simulink model "hoverAlic"  (R2017b)
settings: Solver=VariableStepAuto  StartTime=0.0  StopTime=inf  RelTol=1e-3
values from neighbouring files (symbols this model uses):
  imu = rossubscriber('/imu')    [identification.m]
undefined symbols (not defined in the file or in its folder): Angular, Linear
libraries: robotlib x3, simulink x3
settings Model: Creator=alic  LastModifiedBy=alic

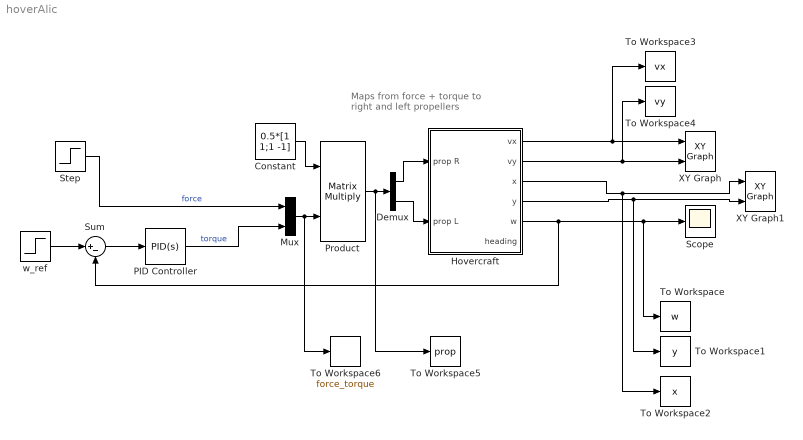
== system hoverAlic ==
  note: Maps from force + torque to
      | right and left propellers
  Constant : Constant  Value=0.5*[1 1;1 -1]
  Demux : Demux  Outputs=2
  Hovercraft : Subsystem
  Mux : Mux  Inputs=2
  PID Controller : simulink/Continuous/PID Controller  Controller=PID  TimeDomain=Continuous-time  SampleTime=-1  IntegratorMethod=Forward Euler  FilterMethod=Forward Euler  Form=Ideal  UseFilter=on  ControllerParametersSource=internal  P=-1.30263726087134  I=1.05750099590497  D=0  N=100  InitialConditionSource=internal  InitialConditionForIntegrator=0  InitialConditionForFilter=0  ExternalReset=none  LimitOutput=off  UpperSaturationLimit=inf  LowerSaturationLimit=-inf  LinearizeAsGain=on  AntiWindupMode=none  Kb=1  TrackingMode=off  Kt=1  PParamMin=[]  PParamMax=[]  IParamMin=[]  IParamMax=[]  DParamMin=[]  DParamMax=[]  NParamMin=[]  NParamMax=[]  KbParamMin=[]  KbParamMax=[]  KtParamMin=[]  KtParamMax=[]  POutMin=[]  POutMax=[]  IOutMin=[]  IOutMax=[]  DOutMin=[]  DOutMax=[]  NOutMin=[]  NOutMax=[]  KbOutMin=[]  KbOutMax=[]  KtOutMin=[]  KtOutMax=[]  IntegratorOutMin=[]  IntegratorOutMax=[]  FilterOutMin=[]  FilterOutMax=[]  SumOutMin=[]  SumOutMax=[]  SumI1OutMin=[]  SumI1OutMax=[]  SumI2OutMin=[]  SumI2OutMax=[]  SumI3OutMin=[]  SumI3OutMax=[]  SumDOutMin=[]  SumDOutMax=[]  SaturationOutMin=[]  SaturationOutMax=[]  IntegratorContinuousStateAttributes=''  IntegratorStateMustResolveToSignalObject=off  IntegratorRTWStateStorageClass=Auto  FilterContinuousStateAttributes=''  FilterStateMustResolveToSignalObject=off  FilterRTWStateStorageClass=Auto  DifferentiatorICPrevScaledInput=0  DifferentiatorOutMin=[]  DifferentiatorOutMax=[]  InitialConditionSetting=State (most efficient)  FilterDiffOutCoefMin=[]  FilterDiffOutCoefMax=[]  SumDenOutMin=[]  SumDenOutMax=[]  SumNumOutMin=[]  SumNumOutMax=[]  ReciprocalOutMin=[]  ReciprocalOutMax=[]  DivideOutMin=[]  DivideOutMax=[]  TunerSelectOption=Transfer Function Based (PID Tuner App)
  Product : Product  Multiplication=Matrix(*)
  Scope : Scope
  Step : Step  After=0.2  SampleTime=3
  Sum : Sum  Inputs=|+-
  To Workspace : ToWorkspace  VariableName=w  SaveFormat=Timeseries  SampleTime=-1
  To Workspace1 : ToWorkspace  VariableName=y  SaveFormat=Timeseries  SampleTime=-1
  To Workspace2 : ToWorkspace  VariableName=x  SaveFormat=Timeseries  SampleTime=-1
  To Workspace3 : ToWorkspace  VariableName=vx  SaveFormat=Timeseries  SampleTime=-1
  To Workspace4 : ToWorkspace  VariableName=vy  SaveFormat=Timeseries  SampleTime=-1
  To Workspace5 : ToWorkspace  VariableName=prop  SaveFormat=Timeseries  SampleTime=-1
  To Workspace6 : ToWorkspace  VariableName=force_torque  SaveFormat=Timeseries  SampleTime=-1
  XY Graph : simulink/Sinks/XY Graph  xmin=-2  xmax=2  ymin=-2  ymax=2  st=-1
  XY Graph1 : simulink/Sinks/XY Graph  xmin=-10  xmax=10  ymin=-10  ymax=10  st=-1
  w_ref : Step  After=0  SampleTime=0
  wires:
  Hovercraft/2(vy) -> To Workspace4/1, XY Graph/2
  Step/1 -> Mux/1  "force"
  Hovercraft/5(w) -> Sum/2, To Workspace/1, Scope/1
  Hovercraft/1(vx) -> To Workspace3/1, XY Graph/1
  Constant/1 -> Product/1
  w_ref/1 -> Sum/1
  Product/1 -> To Workspace5/1, Demux/1
  Mux/1 -> To Workspace6/1, Product/2
  Sum/1 -> PID Controller/1
  Hovercraft/4(y) -> To Workspace1/1, XY Graph1/2
  PID Controller/1 -> Mux/2  "torque"
  Demux/1 -> Hovercraft/1(prop R)
  Hovercraft/3(x) -> To Workspace2/1, XY Graph1/1
  Demux/2 -> Hovercraft/2(prop L)

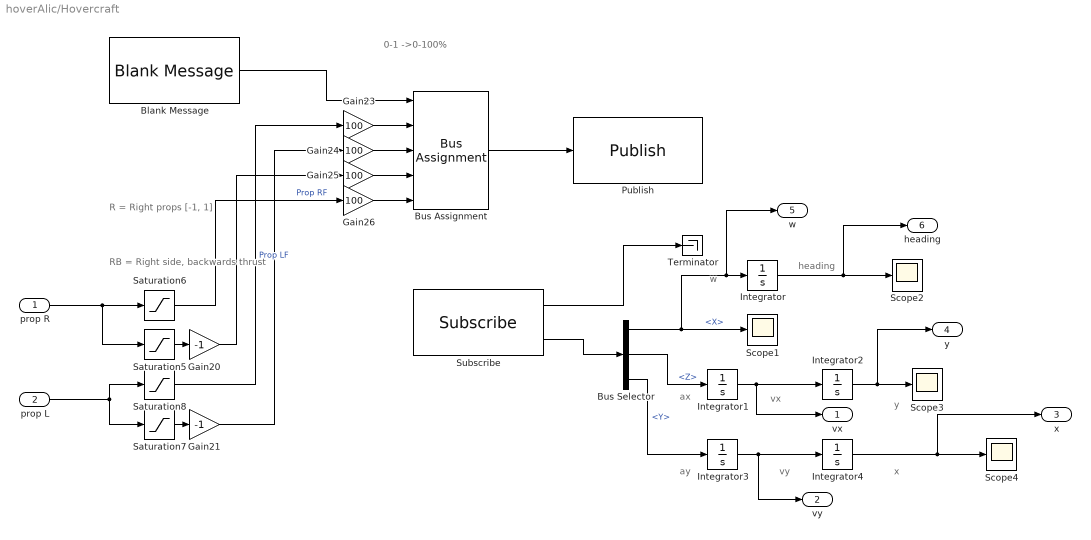
== system hoverAlic/Hovercraft ==
  note: vx
  note: ax
  note: heading
  note: w
  note: 0-1 ->0-100%
  note: R = Right props [-1, 1]
  note: RB = Right side, backwards thrust
  note: ay
  note: vy
  note: x
  note: y
  prop R : Inport
  prop L : Inport  Port=2
  Blank Message : robotlib/Blank Message  SourceLibraryInfo=This block requires Robotics System Toolbox  messageType=geometry_msgs/Twist  SampleTime=inf
      settings: SourceProductBaseCode=RO
  Bus Assignment : BusAssignment  AssignedSignals=Linear.X,Linear.Y,Angular.X,Angular.Y
  Bus Selector : BusSelector  OutputSignals=AngularVelocity.X,LinearAcceleration.Z,LinearAcceleration.Y
  Gain20 : Gain  Gain=-1
  Gain21 : Gain  Gain=-1
  Gain{23..26} (4 alike) : Gain  Gain=100
  Integrator{,1..4} (5 alike) : Integrator
  Publish : robotlib/Publish  SourceLibraryInfo=This block requires Robotics System Toolbox  topicSource=Select from ROS network  topic=/cmd_vel  messageType=geometry_msgs/Twist  messageQueueLength=1
      settings: SourceProductBaseCode=RO
  Saturation5 : Saturate  UpperLimit=0  LowerLimit=-1
  Saturation6 : Saturate  UpperLimit=1  LowerLimit=0
  Saturation7 : Saturate  UpperLimit=0  LowerLimit=-1
  Saturation8 : Saturate  UpperLimit=1  LowerLimit=0
  Scope{1..4} (4 alike) : Scope
  Subscribe : robotlib/Subscribe  SourceLibraryInfo=This block requires Robotics System Toolbox  topicSource=Select from ROS network  topic=/imu  messageType=sensor_msgs/Imu  sampleTime=-1  messageQueueLength=1
      settings: SourceProductBaseCode=RO
  Terminator : Terminator
  vx : Outport
  vy : Outport  Port=2
  x : Outport  Port=3
  y : Outport  Port=4
  w : Outport  Port=5
  heading : Outport  Port=6
  wires:
  Integrator3/1 -> vy/1, Integrator4/1
  Integrator2/1 -> y/1, Scope3/1
  Bus Selector/3 -> Integrator3/1  "<Y>"
  Integrator1/1 -> vx/1, Integrator2/1
  Integrator/1 -> heading/1, Scope2/1
  Bus Selector/2 -> Integrator1/1  "<Z>"
  Bus Selector/1 -> w/1, Integrator/1, Scope1/1  "<X>"
  Bus Assignment/1 -> Publish/1
  Saturation7/1 -> Gain21/1
  Gain21/1 -> Gain24/1
  Gain23/1 -> Bus Assignment/2
  Gain26/1 -> Bus Assignment/5
  Subscribe/1 -> Terminator/1
  Gain20/1 -> Gain25/1
  Saturation6/1 -> Gain26/1  "Prop RF"
  Saturation8/1 -> Gain23/1  "Prop LF"
  Subscribe/2 -> Bus Selector/1
  Gain25/1 -> Bus Assignment/4
  Blank Message/1 -> Bus Assignment/1
  Gain24/1 -> Bus Assignment/3
  Saturation5/1 -> Gain20/1
  prop L/1 -> Saturation7/1, Saturation8/1
  Integrator4/1 -> x/1, Scope4/1
  prop R/1 -> Saturation5/1, Saturation6/1
